simulink model "Particulas"  (R2020b)
settings: Solver=ode45  StartTime=0.0  StopTime=200  FixedStep=1e-7  RelTol=1e-4  AbsTol=1e-4  EnableMultiTasking=on
settings Model: EnablePacing=on  PacingRate=0.500000  Creator=André  LastModifiedBy=Andre
settings SolverCC: AutoScaleAbsTol=off  ConsecutiveZCsStepRelTol=100*128*eps  ShapePreserveControl=EnableAll  ZeroCrossControl=EnableAll  AutoInsertRateTranBlk=on
settings DataIOCC: LimitDataPoints=on  SaveFormat=Array  SignalLoggingSaveFormat=ModelDataLogs  ReturnWorkspaceOutputs=off
settings OptimizationCC: ExpressionDepthLimit=2147483647  LifeSpan=inf
settings DebuggingCC: UnderspecifiedInitializationDetection=Classic  MergeDetectMultiDrivingBlocksExec=none  SolverPrmCheckMsg=warning  FcnCallInpInsideContextMsg=warning  StateNameClashWarn=warning  SFUnexpectedBacktrackingDiag=warning  SFNoUnconditionalDefaultTransitionDiag=warning  SFExecutionAtInitializationDiag=none  ArithmeticOperatorsInVariantConditions=warning
settings HardwareCC: ProdBitPerPointer=32  ProdBitPerSizeT=32  ProdBitPerPtrDiffT=32  ProdLargestAtomicFloat=None  ProdIntDivRoundTo=Undefined  ProdEndianess=Unspecified  ProdWordSize=32  ProdHWDeviceType=32-bit Generic
settings ModelReferenceCC: PropagateSignalLabelsOutOfModel=off
settings SFSimCC: SimUseLocalCustomCode=off  SimParseCustomCode=off  CustomCodeUndefinedFunction=UseInterfaceOnly
settings RTWCC: RTWUseLocalCustomCode=off
settings CodeAppCC: StateflowObjectComments=on
settings GRTTargetCC: TargetLangStandard=C89/C90 (ANSI)  CombineOutputUpdateFcns=off  GRTInterface=on
settings ConfigComp: CovMetricSettings=dw  CovSaveCumulativeToWorkspaceVar=on  CovSaveSingleToWorkspaceVar=on  CovExternalEMLEnable=off

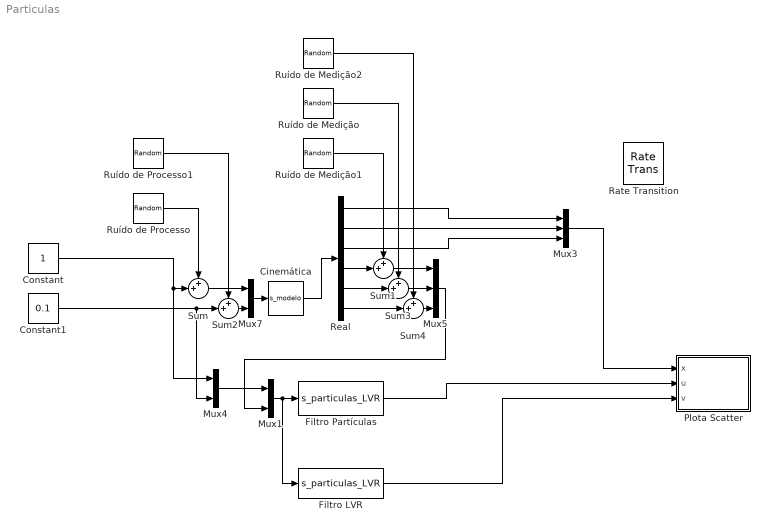
== system Particulas ==
  Cinemática : S-Function  FunctionName=s_modelo  Parameters=[1 -5 0]  SFunctionDeploymentMode=off  EnableBusSupport=off
  Constant : Constant
  Constant1 : Constant  Value=0.1
  Filtro LVR : S-Function  FunctionName=s_particulas_LVR  Parameters=[0 -6 0 1 1]  SFunctionDeploymentMode=off  EnableBusSupport=off
  Filtro Partículas : S-Function  FunctionName=s_particulas_LVR  Parameters=[0 -6 0 0 1]  SFunctionDeploymentMode=off  EnableBusSupport=off
  Mux1 : Mux  Inputs=2
  Mux3 : Mux  Inputs=3
  Mux4 : Mux  Inputs=2
  Mux5 : Mux  Inputs=3
  Mux7 : Mux  Inputs=2
  Plota Scatter : MATLAB Function  TreatAsAtomicUnit=on
  Rate Transition : RateTransition  OutPortSampleTime=1
  Real : Demux  Outputs=6
  Ruído de Medição : RandomNumber  Variance=0.1  SampleTime=0.01
  Ruído de Medição1 : RandomNumber  Variance=0.1  SampleTime=0.01
  Ruído de Medição2 : RandomNumber  Variance=0.1  SampleTime=0.01
  Ruído de Processo : RandomNumber  Variance=0.1  SampleTime=0.1
  Ruído de Processo1 : RandomNumber  Variance=0.1  SampleTime=0.1
  Sum{,1..4} (5 alike) : Sum  Inputs=++|
  wires:
  Mux1/1 -> Filtro LVR/1, Filtro Partículas/1
  Mux7/1 -> Cinemática/1
  Mux5/1 -> Mux1/2
  Sum2/1 -> Mux7/2
  Constant/1 -> Mux4/1, Sum/2
  Sum/1 -> Mux7/1
  Mux4/1 -> Mux1/1
  Cinemática/1 -> Real/1
  Sum4/1 -> Mux5/3
  Constant1/1 -> Mux4/2, Sum2/2
  Real/6 -> Sum4/2
  Real/5 -> Sum3/2
  Real/4 -> Sum1/2
  Real/1 -> Mux3/1
  Real/2 -> Mux3/2
  Sum3/1 -> Mux5/2
  Sum1/1 -> Mux5/1
  Ruído de Processo/1 -> Sum/1
  Filtro Partículas/1 -> Plota Scatter/2(u)
  Filtro LVR/1 -> Plota Scatter/3(v)
  Ruído de Medição2/1 -> Sum4/1
  Ruído de Medição/1 -> Sum3/1
  Ruído de Medição1/1 -> Sum1/1
  Ruído de Processo1/1 -> Sum2/1
  Mux3/1 -> Plota Scatter/1(x)
  Real/3 -> Mux3/3

== matlab function Particulas/Plota Scatter ==
  data: x input; u input; v input
function  fcn(x,u,v)
     %n_Particulas = 1000;  
     marker = [0 0; 5 5; 0 5]; % Positions of markers
     eixos =[-50 50 -50 50];
     %n_estados = n_Particulas*3;

     coder.extrinsic('scatter')
     coder.extrinsic('subplot')
     coder.extrinsic('quiver')
     subplot(2,1,1);
      particulas = u(:);
      xP = reshape(particulas,4,[]);
      x_ = mean(xP(1:3,:).*([1 1 1]'*xP(4,:)), 2)/mean(xP(4,:));
      scatter(xP(1,:),xP(2,:), 'k.');
      axis( eixos);
      grid on;
      hold on;
      title('PF');
      scatter(x_(1),x_(2),'bo');
      quiver(x_(1),x_(2),cos(x_(3)),sin(x_(3)),5,'Color','b','LineWidth',0.5,'MaxHeadSize',0.4);
      scatter(marker(:,1),marker(:,2), 'gs');
      scatter(x(1),x(2), 'r*');
      quiver(x(1),x(2),cos(x(3)),sin(x(3)),5,'Color','r','LineWidth',0.5,'MaxHeadSize',0.4);
      hold off;

     subplot(2,1,2);
      particulas = v(:);
      xP = reshape(particulas,4,[]);
      x_ = mean(xP(1:3,:).*([1 1 1]'*xP(4,:)), 2)/mean(xP(4,:));
      scatter(xP(1,:),xP(2,:), 'k.');
      axis( eixos);
      grid on;
      hold on;
      title('PF - LVR');
      quiver(x_(1),x_(2),cos(x_(3)),sin(x_(3)),5,'Color','b','LineWidth',0.5,'MaxHeadSize',0.4);
      scatter(marker(:,1),marker(:,2), 'gs');
      scatter(x(1),x(2), 'r*');
      quiver(x(1),x(2),cos(x(3)),sin(x(3)),5,'Color','r','LineWidth',0.5,'MaxHeadSize',0.4);
      hold off;
     % insert additional code as needed to turn on grid, setup axis limits, etc.

  %%%%%%%%%
%y = u;
